simulink model "ch5example5"  (Simulink 5.0)
settings: Solver=ode5  StartTime=0.0  StopTime=10.0  FixedStep=1/1e6  RelTol=1e-3
undefined symbols (not defined in the file): get
libraries: dsparch4 x2, dspsnks4 x1, commcontsrc2 x1
settings Model: LastModifiedBy=shaoyubin

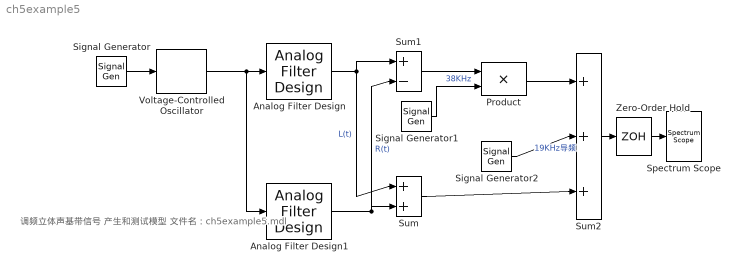
== system ch5example5 ==
  note: 调频立体声基带信号
      | 产生和测试模型
      | 文件名：ch5example5.mdl
  Analog Filter Design : dsparch4/Analog Filter Design  method=Butterworth  filttype=Bandpass  N=1  Wlo=2*pi*1500  Whi=2*pi*15e3  Rp=2  Rs=40
  Analog Filter Design1 : dsparch4/Analog Filter Design  method=Butterworth  filttype=Lowpass  N=1  Wlo=2*pi*5e3  Whi=2*pi*10e3  Rp=2  Rs=40
  Product : Product  SaturateOnIntegerOverflow=on
  Signal Generator : SignalGenerator  Frequency=10
  Signal Generator1 : SignalGenerator  Frequency=38e3
  Signal Generator2 : SignalGenerator  Frequency=19e3
  Spectrum Scope : dspsnks4/Spectrum Scope  ScopeProperties=off  Domain=Frequency  HorizSpan=1  UseBuffer=on  BufferSize=1024  Overlap=512  inpFftLenInherit=on  FFTlength=512  numAvg=2  DisplayProperties=on  AxisGrid=on  Memory=off  FrameNumber=on  AxisLegend=off  AxisZoom=off  OpenScopeAtSimStart=on  OpenScopeImmediately=off  FigPos=get(0,'defaultfigureposition')  AxisProperties=off  XUnits=Hertz  XRange=[0...Fs/2]  InheritXIncr=on  XIncr=1.0  XLabel=Samples  YUnits=Magnitude  YLabel=Magnitude  LineProperties=off
      settings: YMin=-2.83974209799737  YMax=59.776604918878
  Sum : Sum  Inputs=|++  SaturateOnIntegerOverflow=on
  Sum1 : Sum  Inputs=|+-  SaturateOnIntegerOverflow=on
  Sum2 : Sum  Inputs=|+++  SaturateOnIntegerOverflow=on
  Voltage-Controlled Oscillator : commcontsrc2/Voltage-Controlled Oscillator  Ac=1  Fc=(500+15e3)/2  Kc=((500+15e3)/2-500)  Ph=0
  Zero-Order Hold : ZeroOrderHold  SampleTime=0.5e-5
  wires:
  Zero-Order Hold/1 -> Spectrum Scope/1
  Signal Generator/1 -> Voltage-Controlled Oscillator/1
  Analog Filter Design1/1 -> Sum/2, Sum1/2  "R(t)"
  Analog Filter Design/1 -> Sum/1, Sum1/1  "L(t)"
  Sum1/1 -> Product/1
  Signal Generator1/1 -> Product/2  "38KHz"
  Product/1 -> Sum2/1
  Signal Generator2/1 -> Sum2/2  "19KHz导频"
  Sum/1 -> Sum2/3
  Sum2/1 -> Zero-Order Hold/1
  Voltage-Controlled Oscillator/1 -> Analog Filter Design/1, Analog Filter Design1/1
